simulink model "Mechanical_Model"  (R2023b)
settings: Solver=VariableStepAuto  StartTime=0.0  StopTime=50  RelTol=1e-3
values from neighbouring files (symbols this model uses):
  A = M1^(-1)*M2    [QUBE2_Control_System.m]    (also in QUBE2_Mechanical_Formulation.m = double(subs(A,[Lr lp Jr_ex mp Jp g Ke Kc Ra Br Bp],[Lr_ lp_ )
  alpha_0 = 0    [QUBE2_Mechanical_Formulation.m]
  B = M1^(-1)*M3    [QUBE2_Control_System.m]    (also in QUBE2_Mechanical_Formulation.m = double(subs(B,[Lr lp Jr_ex mp Jp g Ke Kc Ra Br Bp],[Lr_ lp_ )
  C = [1,0,0,0 ... (first row only)    [QUBE2_Control_System.m]    (also in QUBE2_Mechanical_Formulation.m)
  D = 0    [QUBE2_Control_System.m]    (also in QUBE2_Mechanical_Formulation.m = [0)
  g_ = 9.81    [QUBE2_Mechanical_Formulation.m]
  Jp_ = (1/12)*mp_*(3*rp^2 + Lp^2)    (= 3.3718538025e-05)    [QUBE2_Mechanical_Formulation.m]
  Jr_ex_ = 9e-5    (= 9e-05)    [QUBE2_Mechanical_Formulation.m]
  K = [0, 0; 0, g*l1*m1]    [QUBE2_Control_System.m]    (also in QUBE2_Mechanical_Formulation.m = place(A,B,P))
  Kc_ = 0.042    [QUBE2_Mechanical_Formulation.m]
  Ke_ = 0.042    [QUBE2_Mechanical_Formulation.m]
  lp_ = 0.95*Lp/2    (= 0.061275)    [QUBE2_Mechanical_Formulation.m]
  Lr_ = 0.09    [QUBE2_Mechanical_Formulation.m]
  mp_ = 0.02421    [QUBE2_Mechanical_Formulation.m]
  Ra_ = 8.4    [QUBE2_Mechanical_Formulation.m]
  theta_0 = 0    [QUBE2_Mechanical_Formulation.m]
  Va_0 = 0    [QUBE2_Mechanical_Formulation.m]
libraries: simulink_extras x2
settings Model: Creator=mozar  LastModifiedBy=mozar

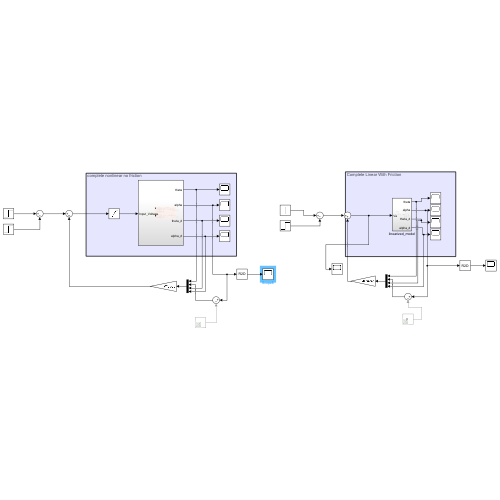
[thumbnail: Simulink's stored preview of the top-level diagram]
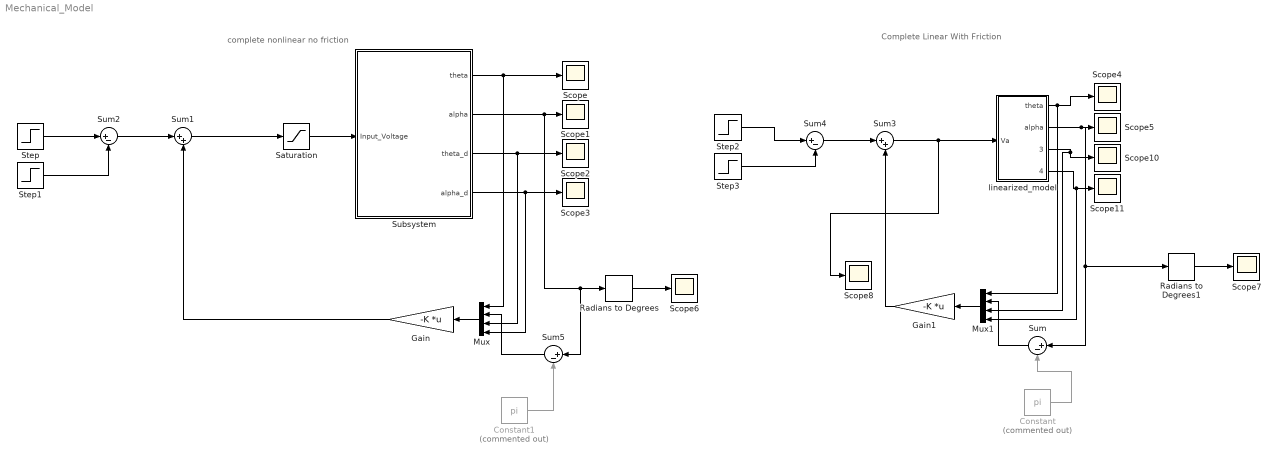
== system Mechanical_Model ==
  note: Complete Linear With Friction
  note: complete nonlinear no friction
  Constant : Constant  Commented=on  Value=pi
  Constant1 : Constant  Commented=on  Value=pi
  Gain : Gain  Gain=-K  Multiplication=Matrix(K*u) (u vector)
  Gain1 : Gain  Gain=-K  Multiplication=Matrix(K*u) (u vector)
  Mux : Mux
  Mux1 : Mux
  Radians to Degrees : simulink_extras/Transformations/Radians to Degrees
  Radians to Degrees1 : simulink_extras/Transformations/Radians to Degrees
  Saturation : Saturate  UpperLimit=10  LowerLimit=-10
  Scope{,1..8,10..11} (11 alike) : Scope
  Step : Step  SampleTime=0
  Step1 : Step  Time=1.05  Before=1  SampleTime=0
  Step2 : Step  After=5  SampleTime=0
  Step3 : Step  Time=1.05  Before=1  After=5  SampleTime=0
  Subsystem : Subsystem
  Sum{,2,4..5} (4 alike) : Sum  Inputs=|+-
  Sum1 : Sum  Inputs=|++
  Sum3 : Sum  Inputs=|++
  linearized_model : Subsystem
  wires:
  Subsystem/1(theta) -> Mux/1, Scope/1
  Subsystem/2(alpha) -> Sum5/1, Radians to Degrees/1, Scope1/1
  linearized_model/2(alpha) -> Sum/1, Radians to Degrees1/1, Scope5/1
  Subsystem/3(theta_d) -> Mux/3, Scope2/1
  linearized_model/4(alpha_d) -> Mux1/4, Scope11/1
  linearized_model/1(theta) -> Mux1/1, Scope4/1
  linearized_model/3(theta_d) -> Mux1/3, Scope10/1
  Subsystem/4(alpha_d) -> Mux/4, Scope3/1
  Saturation/1 -> Subsystem/1(Input_Voltage)
  Sum2/1 -> Sum1/1
  Step/1 -> Sum2/1
  Step1/1 -> Sum2/2
  Radians to Degrees/1 -> Scope6/1
  Sum1/1 -> Saturation/1
  Mux/1 -> Gain/1
  Gain/1 -> Sum1/2
  Mux1/1 -> Gain1/1
  Gain1/1 -> Sum3/2
  Step2/1 -> Sum4/1
  Step3/1 -> Sum4/2
  Sum4/1 -> Sum3/1
  Sum3/1 -> Scope8/1, linearized_model/1(Va)
  Radians to Degrees1/1 -> Scope7/1
  Sum/1 -> Mux1/2
  Constant/1 -> Sum/2
  Sum5/1 -> Mux/2
  Constant1/1 -> Sum5/2

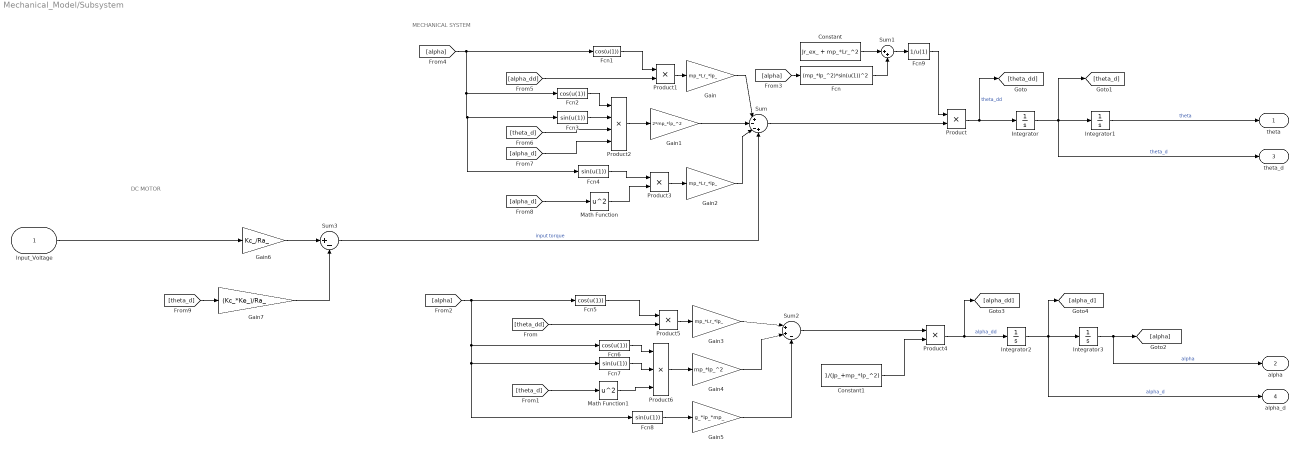
== system Mechanical_Model/Subsystem ==
  note: DC MOTOR
  note: MECHANICAL SYSTEM
  Input_Voltage : Inport
  Constant : Constant  Value=Jr_ex_ + mp_*Lr_^2
  Constant1 : Constant  Value=1/(Jp_+mp_*lp_^2)
  Fcn : Fcn  Expr=(mp_*lp_^2)*sin(u(1))^2
  Fcn{1..2,5..6} (4 alike) : Fcn  Expr=cos(u(1))
  Fcn{3..4,7..8} (4 alike) : Fcn  Expr=sin(u(1))
  Fcn9 : Fcn  Expr=1/u(1)
  Gain : Gain  Gain=mp_*Lr_*lp_
  Gain1 : Gain  Gain=2*mp_*lp_^2
  Gain2 : Gain  Gain=mp_*Lr_*lp_
  Gain3 : Gain  Gain=mp_*Lr_*lp_
  Gain4 : Gain  Gain=mp_*lp_^2
  Gain5 : Gain  Gain=g_*lp_*mp_
  Gain6 : Gain  Gain=Kc_/Ra_
  Gain7 : Gain  Gain=(Kc_*Ke_)/Ra_
  Integrator{,1..3} (4 alike) : Integrator
  Math Function : Math  Operator=square
  Math Function1 : Math  Operator=square
  Product{,1,3..5} (5 alike) : Product
  Product2 : Product  Inputs=4
  Product6 : Product  Inputs=3
  Sum : Sum  Inputs=|+--+
  Sum1 : Sum  Inputs=|++
  Sum2 : Sum  Inputs=|++-
  Sum3 : Sum  Inputs=|+-
  theta : Outport
  alpha : Outport  Port=2
  theta_d : Outport  Port=3
  alpha_d : Outport  Port=4
  wires:
  Integrator2/1 -> alpha_d/1, Integrator3/1, [alpha_d]  "alpha_d"
  Fcn6/1 -> Product6/1
  Product4/1 -> [alpha_dd], Integrator2/1  "alpha_dd"
  Fcn4/1 -> Product3/1
  Integrator/1 -> theta_d/1, [theta_d], Integrator1/1  "theta_d"
  Gain1/1 -> Sum/2
  Gain6/1 -> Sum3/1
  Fcn3/1 -> Product2/2
  Fcn1/1 -> Product1/1
  Integrator1/1 -> theta/1  "theta"
  Fcn8/1 -> Gain5/1
  Fcn7/1 -> Product6/2
  Gain5/1 -> Sum2/3
  Sum1/1 -> Fcn9/1
  Fcn/1 -> Sum1/2
  Product1/1 -> Gain/1
  Fcn9/1 -> Product/1
  Product3/1 -> Gain2/1
  Sum/1 -> Product/2
  [alpha_d] -> Math Function/1
  [theta_dd] -> Product5/2
  [theta_d] -> Gain7/1
  Product5/1 -> Gain3/1
  Integrator3/1 -> alpha/1, [alpha]  "alpha"
  Fcn5/1 -> Product5/1
  Product6/1 -> Gain4/1
  Sum2/1 -> Product4/1
  Math Function1/1 -> Product6/3
  Math Function/1 -> Product3/2
  Product/1 -> Integrator/1, [theta_dd]  "theta_dd"
  Gain4/1 -> Sum2/2
  Input_Voltage/1 -> Gain6/1
  Constant/1 -> Sum1/1
  [alpha] -> Fcn8/1, Fcn7/1, Fcn6/1, Fcn5/1
  Constant1/1 -> Product4/2
  Product2/1 -> Gain1/1
  [alpha] -> Fcn4/1, Fcn3/1, Fcn2/1, Fcn1/1
  [alpha_d] -> Product2/4
  [alpha_dd] -> Product1/2
  [alpha] -> Fcn/1
  Fcn2/1 -> Product2/1
  Sum3/1 -> Sum/4  "input torque"
  Gain2/1 -> Sum/3
  Gain/1 -> Sum/1
  Gain3/1 -> Sum2/1
  [theta_d] -> Math Function1/1
  Gain7/1 -> Sum3/2
  [theta_d] -> Product2/3

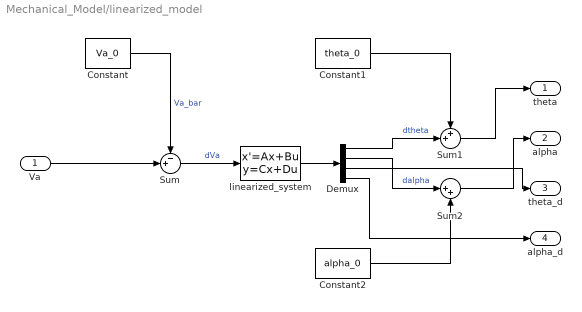
== system Mechanical_Model/linearized_model ==
  Va : Inport
  Constant : Constant  Value=Va_0
  Constant1 : Constant  Value=theta_0
  Constant2 : Constant  Value=alpha_0
  Demux : Demux
  Sum : Sum  Inputs=-+|
  Sum1 : Sum  Inputs=++|
  Sum2 : Sum  Inputs=|++
  linearized_system : StateSpace  A=A  B=B  C=C  D=D  InitialCondition=0
  theta : Outport
  alpha : Outport  Port=2
  theta_d : Outport  Port=3
  alpha_d : Outport  Port=4
  wires:
  Va/1 -> Sum/2
  Demux/1 -> Sum1/2  "dtheta"
  linearized_system/1 -> Demux/1
  Constant/1 -> Sum/1  "Va_bar"
  Sum/1 -> linearized_system/1  "dVa"
  Constant1/1 -> Sum1/1
  Constant2/1 -> Sum2/2
  Sum2/1 -> alpha/1
  Demux/2 -> Sum2/1  "dalpha"
  Sum1/1 -> theta/1
  Demux/3 -> theta_d/1
  Demux/4 -> alpha_d/1
